simulink model "EcoSIM3_P2_C2_WIP"  (R2014b)
settings: Solver=ode1  SolverMode=SingleTasking  StartTime=0.0  StopTime=inf  FixedStep=0.01  RelTol=1e-3
PostLoadFcn:
  | %, if any(exist('dsrtsu_mdlpostloadfcn', 'file') == [2, 3, 6]), try dsrtsu_mdlpostloadfcn('Execute', bdroot); catch fprintf('Error in PostLoadFcn (dsrtsu_mdlpostloadfcn) for model "%s":\n %s\n', bdroot, lasterr); end, end,
InitFcn:
  | tic
  | %Startup_EcoSIM
values from neighbouring files (symbols this model uses):
  EngPwr = [0 5	10	15	20	25	30	35	40	45	50	55	60	65	70	75	80	85	90	95	100	105	110	115]    [Series_Maps.m]
  EngSpd = [0 477.4645 954.929 1909.858 2864.787 3819.716 4774.645 5729.574 6684.503]    [Series_Maps.m]
  EngTrq = [0	0	0	0	0	0	0	0	0	0	0	0	0	0	0	0	0	0	0	0	0	0	0	0 ... (first row only)    [Series_Maps.m]
  Power = [0 5 10 15 20 25 30]    [Series_Maps.m]
  Torque = [-50,-40,-30,-25,-20,-15,-10,-8,-6,-4,-2,0]    [Series_Maps.m]
undefined symbols (not defined in the file or in its folder): canChannel, Controls, DriveCycles, Driver, EM_EFF_MAP, EM_PwrLoss_MAP, Glbl, Overwritten_Mode, Plants, sigbuilder_block, Trialmap, Veh_Dynamics
libraries: simulink x141, canmsglib x113, fl_lib x104, canlib x89, nesl_utility x56, sdl_lib x29, dspsigops x6, dspswit3 x5, dspstat3 x2, commnoisgen2 x1, dspfdesign x1
(part 19 of 21)

== system EcoSIM3_P2_C2_WIP/Supervisory Controller/Functional Safety1/Functional Safety Algorithm/Fault Detection (Team Developed)/Torque Security Faults/Torque Estimation/Electric Motor Torque Estimation ==
  In1 : Inport
  Bus Selector : BusSelector  OutputSignals=Vehicle_Speed_meter_per_s,ESS_Transmit.bcm_vbat,ESS_Transmit.bcm_ibat,BAS_Transmit.BAS_Speed_rad_per_s,BAS_Transmit.BAS_Torque_Command_Nm
  EM DC Current Est : Subsystem
  EM Speed Est : Subsystem
  EM Torque Est : Subsystem
  Out1 : Outport
  wires:
  EM Torque Est/1(EM Trq Est [Nm]) -> Out1/1
  EM DC Current Est/1(EM DC Current Est [A]) -> EM Torque Est/3(EM DC Current Est [A])
  EM Speed Est/1(EM Speed Est [rad/s]) -> EM Torque Est/1(EM Speed [rad/s])
  Bus Selector/5 -> EM DC Current Est/4(BAS Torque [Nm])  "<BAS_Torque_Command_Nm>"
  Bus Selector/4 -> EM DC Current Est/3(BAS Speed [rad/s])  "<BAS_Speed_rad_per_s>"
  Bus Selector/3 -> EM DC Current Est/2(Batt Current [A])  "<bcm_ibat>"
  Bus Selector/2 -> EM Torque Est/2(Batt Voltage [V]), EM DC Current Est/1(Batt Voltage [V])  "<bcm_vbat>"
  Bus Selector/1 -> EM Speed Est/1(Vehicle Speed [m/s])  "<Vehicle_Speed_meter_per_s>"
  In1/1 -> Bus Selector/1

== system EcoSIM3_P2_C2_WIP/Supervisory Controller/Functional Safety1/Functional Safety Algorithm/Fault Detection (Team Developed)/Torque Security Faults/Torque Estimation/Engine Torque Estimation ==
  In1 : Inport
  Out1 : Outport

== system EcoSIM3_P2_C2_WIP/Supervisory Controller/Functional Safety1/Functional Safety Algorithm/Fault Detection (Team Developed)/Torque Security Faults/Torque Estimation/PTU Torque Estimation ==
  In1 : Inport
  Out1 : Outport

== system EcoSIM3_P2_C2_WIP/Supervisory Controller/Functional Safety1/Functional Safety Algorithm/Fault Detection (Team Developed)/Torque Security Faults/Torque Estimation/Rear Diff Torque Estimation ==
  In1 : Inport
  Out1 : Outport

== system EcoSIM3_P2_C2_WIP/Supervisory Controller/Functional Safety1/Functional Safety Algorithm/Fault Detection (Team Developed)/Torque Security Faults/Torque Estimation/Trans Torque Estimation ==
  In1 : Inport
  Out1 : Outport

== system EcoSIM3_P2_C2_WIP/Supervisory Controller/Functional Safety1/Functional Safety Algorithm/Fault Detection (Team Developed)/Torque Security Faults/Torque Estimation/Wheel Torque Estimation ==
  Veh Mass Est : Inport
  ECU/Sensor Signals : Inport  Port=2
  Bus Selector : BusSelector  OutputSignals=Vehicle_Speed_meter_per_s
  Derivative : Derivative
  Product : Product
  Product1 : Product
  Wheel Radius : Constant  Value=Plants.Rear_wh.tire_diameter/2
  Whl Trq Est : Outport
  wires:
  Bus Selector/1 -> Derivative/1  "<Vehicle_Speed_meter_per_s>"
  Derivative/1 -> Product/2  "Veh_Accel"
  Product1/1 -> Whl Trq Est/1  "Whl_Trq_Est_Nm"
  Wheel Radius/1 -> Product1/2
  Product/1 -> Product1/1
  ECU/Sensor Signals/1 -> Bus Selector/1
  Veh Mass Est/1 -> Product/1

== system EcoSIM3_P2_C2_WIP/Supervisory Controller/Functional Safety1/Functional Safety Algorithm/Fault Detection (Team Developed)/Torque Security Faults/Vehicle Mass Estimation/Belt Coupler ==
  BAS Torque : Inport
  Proportional Gain : Gain  Gain=Plants.Belt.GR
  Proportional Gain1 : Gain  Gain=Plants.Belt.GR
  Out1 : Outport
  wires:
  BAS Torque/1 -> Proportional Gain1/1
  Proportional Gain1/1 -> Proportional Gain/1
  Proportional Gain/1 -> Out1/1

== system EcoSIM3_P2_C2_WIP/Supervisory Controller/Functional Safety1/Functional Safety Algorithm/Fault Detection (Team Developed)/Torque Security Faults/Vehicle Mass Estimation/Driveline ==
  EM_Torque : Inport
  Mechanical Coupler : Subsystem
  Rear Diff : Subsystem
  Rear Wheels : Subsystem
  Out1 : Outport
  wires:
  Rear Wheels/1(Out1) -> Out1/1
  EM_Torque/1 -> Mechanical Coupler/1(In1)
  Mechanical Coupler/1(Out1) -> Rear Diff/1(In1)
  Rear Diff/1(Out1) -> Rear Wheels/1(In1)

== system EcoSIM3_P2_C2_WIP/Supervisory Controller/Functional Safety1/Functional Safety Algorithm/Fault Detection (Team Developed)/Torque Security Faults/Vehicle Mass Estimation/Driveline1 ==
  In1 : Inport
  Mechanical Coupler : Subsystem
  Rear Diff : Subsystem
  Rear Wheels : Subsystem
  Out1 : Outport
  wires:
  Rear Diff/1(Out1) -> Rear Wheels/1(In1)
  Mechanical Coupler/1(Out1) -> Rear Diff/1(In1)
  In1/1 -> Mechanical Coupler/1(In1)
  Rear Wheels/1(Out1) -> Out1/1

== system EcoSIM3_P2_C2_WIP/Supervisory Controller/Functional Safety1/Functional Safety Algorithm/Fault Detection (Team Developed)/Torque Security Faults/Vehicle Mass Estimation/Driveline2 ==
  In1 : Inport
  Mechanical Coupler : Subsystem
  Rear Diff : Subsystem
  Rear Wheels : Subsystem
  Out1 : Outport
  wires:
  Rear Wheels/1(Out1) -> Out1/1
  In1/1 -> Mechanical Coupler/1(In1)
  Mechanical Coupler/1(Out1) -> Rear Diff/1(In1)
  Rear Diff/1(Out1) -> Rear Wheels/1(In1)

== system EcoSIM3_P2_C2_WIP/Supervisory Controller/Functional Safety1/Functional Safety Algorithm/Fault Detection (Team Developed)/Torque Security Faults/Vehicle Mass Estimation/Resistance Forces ==
  Vehicle_Speed [m/s] : Inport
  Grade [%] : Inport  Port=2
  Vehicle_Mass [kg] : Inport  Port=3
  Aerodynamic Drag Function : Fcn  Expr=0.5*Glbl.den_air*Veh_Dynamics.Body.Aero_Drag_Coeff*Veh_Dynamics.Body.Frontal_Area*u^2
  Gain : Gain  Gain=Glbl.perc_to_frac
  Grade Resistance Function : Fcn  Expr=Glbl.g*sin(u)
  Percent Grade to Radians : Trigonometry  Operator=atan
  Product1 : Product  Inputs=**  RndMeth=Zero
  Rolling Resistance Function : Subsystem
  Sum1 : Sum  Inputs=+++  SaturateOnIntegerOverflow=on  InputSameDT=on  OutDataTypeStr=Inherit: Same as first input
  Road_Load_Force [N] : Outport
  wires:
  Grade [%]/1 -> Gain/1
  Gain/1 -> Percent Grade to Radians/1
  Vehicle_Mass [kg]/1 -> Product1/2, Rolling Resistance Function/1(Mass)
  Sum1/1 -> Road_Load_Force [N]/1  "Road_Load_Force_N"
  Vehicle_Speed [m/s]/1 -> Rolling Resistance Function/2(Vehicle Speed), Aerodynamic Drag Function/1
  Aerodynamic Drag Function/1 -> Sum1/1
  Grade Resistance Function/1 -> Product1/1
  Product1/1 -> Sum1/2
  Percent Grade to Radians/1 -> Rolling Resistance Function/3(Grade), Grade Resistance Function/1
  Rolling Resistance Function/1(Out2) -> Sum1/3

== system EcoSIM3_P2_C2_WIP/Supervisory Controller/Functional Safety1/Functional Safety Algorithm/Fault Detection (Team Developed)/Torque Security Faults/Vehicle Mass Estimation/Trans ==
  Current Gear : Inport
  ICE_Torque : Inport  Port=2
  Efficiency : Gain  Gain=Plants.Clutch.Eff
  Negative Torque : Gain  Gain=1/Plants.Trans.Mdl.Plant.eff  SaturateOnIntegerOverflow=on  OutDataTypeStr=Inherit: Same as input  ParamDataTypeStr=Inherit: Same as input
  Positive Torque : Gain  Gain=Plants.Trans.Mdl.Plant.eff  SaturateOnIntegerOverflow=on  OutDataTypeStr=Inherit: Same as input  ParamDataTypeStr=Inherit: Same as input
  Product1 : Product  SaturateOnIntegerOverflow=on  InputSameDT=on  OutDataTypeStr=Inherit: Same as first input
  Switch : Switch  SaturateOnIntegerOverflow=on  InputSameDT=on
  Trams GR : Lookup  InputValues=Plants.Trans.Mdl.Plant.Gear_cmd  Table=Plants.Trans.Mdl.Plant.GR  LookUpMeth=Use Input Nearest
  Out1 : Outport
  wires:
  Current Gear/1 -> Trams GR/1
  Switch/1 -> Out1/1  "Trans_Torque_Out_Nm"
  ICE_Torque/1 -> Efficiency/1
  Efficiency/1 -> Product1/2
  Product1/1 -> Switch/2, Positive Torque/1, Negative Torque/1
  Positive Torque/1 -> Switch/1
  Negative Torque/1 -> Switch/3
  Trams GR/1 -> Product1/1  "Trans_GR_Out"

== system EcoSIM3_P2_C2_WIP/Supervisory Controller/Functional Safety1/Functional Safety Algorithm/Fault Detection (Team Developed)/Torque Security Faults/Vehicle Mass Estimation/Trans1 ==
  Current Gear : Inport
  In1 : Inport  Port=2
  Efficiency : Gain  Gain=Plants.Clutch.Eff
  Negative Torque : Gain  Gain=1/Plants.Trans.Mdl.Plant.eff  SaturateOnIntegerOverflow=on  OutDataTypeStr=Inherit: Same as input  ParamDataTypeStr=Inherit: Same as input
  Positive Torque : Gain  Gain=Plants.Trans.Mdl.Plant.eff  SaturateOnIntegerOverflow=on  OutDataTypeStr=Inherit: Same as input  ParamDataTypeStr=Inherit: Same as input
  Product1 : Product  SaturateOnIntegerOverflow=on  InputSameDT=on  OutDataTypeStr=Inherit: Same as first input
  Switch : Switch  SaturateOnIntegerOverflow=on  InputSameDT=on
  Trams GR : Lookup  InputValues=Plants.Trans.Mdl.Plant.Gear_cmd  Table=Plants.Trans.Mdl.Plant.GR  LookUpMeth=Use Input Nearest
  Out1 : Outport
  wires:
  Trams GR/1 -> Product1/1  "Trans_GR_Out"
  Negative Torque/1 -> Switch/3
  Positive Torque/1 -> Switch/1
  Product1/1 -> Negative Torque/1, Positive Torque/1, Switch/2
  Efficiency/1 -> Product1/2
  In1/1 -> Efficiency/1
  Switch/1 -> Out1/1  "Trans_Torque_Out_Nm"
  Current Gear/1 -> Trams GR/1

== system EcoSIM3_P2_C2_WIP/Powertrain/Electrical Storage System/Soft ECU/Algorithm/Current Buffer/Charge Buffer/Moderator-Opposer/Moderator ==
  note: 0.061
  note: 0.1247
  I : Inport
  Compare To Constant : simulink/Logic and Bit Operations/Compare To Constant  relop=>=  const=50  OutDataTypeStr=boolean
  ModeratorHi : Gain  Gain=Plants.ESS.SoftECU.Buffer.Charge.ModeratorHi
  ModeratorLo : Gain  Gain=Plants.ESS.SoftECU.Buffer.Charge.ModeratorLo
  Switch : Switch  Criteria=u2 > Threshold  Threshold=0.5
  O : Outport
  wires:
  I/1 -> ModeratorHi/1, ModeratorLo/1
  ModeratorHi/1 -> Switch/1
  ModeratorLo/1 -> Switch/3
  Switch/1 -> O/1
  [Current] -> Compare To Constant/1
  Compare To Constant/1 -> Switch/2

== system EcoSIM3_P2_C2_WIP/Powertrain/Electrical Storage System/Soft ECU/Algorithm/Current Buffer/Charge Buffer/Moderator-Opposer/Opposer ==
  note: 0.4002
  note: 0.2799
  I : Inport
  Compare To Constant : simulink/Logic and Bit Operations/Compare To Constant  relop=>=  const=50  OutDataTypeStr=boolean
  OpposerHi : Gain  Gain=Plants.ESS.SoftECU.Buffer.Charge.OpposerHi
  OpposerLo : Gain  Gain=Plants.ESS.SoftECU.Buffer.Charge.OpposerLo
  Switch : Switch  Criteria=u2 > Threshold  Threshold=0.5
  O : Outport
  wires:
  [Current] -> Compare To Constant/1
  OpposerLo/1 -> Switch/3
  Compare To Constant/1 -> Switch/2
  OpposerHi/1 -> Switch/1
  Switch/1 -> O/1
  I/1 -> OpposerHi/1, OpposerLo/1

== system EcoSIM3_P2_C2_WIP/Powertrain/Electrical Storage System/Soft ECU/Algorithm/Current Buffer/Discharge Buffer/Moderator-Opposer/Moderator ==
  note: 0.0126
  note: 0.0319
  note: 0.0413
  note: Modeling discharge buffer- Approach 1
      | This model make the assumption that the current required to reduce the buffer is dependent on the current value of the buffer.
      | i.e the current required to cause a further reduction in the buffer when it is at 10% is greater than when it is at 90%. This model
      | multiplies the buffer spent (100- buffer) by a suitable gain (called the Opposer), subtracts it from the current provided by the battery,
      | and the difference is multiplied by a gain (called the Moderator) and integrated to change the buffer. The output of this integrator
      | can be considered as the buffer degradation. Subtracting this from 100 will give us the buffer.
      | Consider an initial buffer of 100%. If a constant current of 50 amps is provided by the battery, the buffer starts reducing, and then
      | reaches an equilibrium point. The buffer reduction rate is higher at the start, then starts reducing as the buffer drop. After reaching the
      | equilibrium point, the buffer remains constant when the current is kept constant. A further increase in current causes the buffer to drop,
      | while a lesser current causes the buffer to rise.
      | Also, it was observed from the dyno data that at a current < 130 amps, the buffer behaviour depends on the value of the current, while
      | at currents over 130 amps, the drop is independent of the current magnitude. Also, if the current exceeeds 340 amps, the buffer reduction
      | rate steepens.
      | Using the data from dyno testing, the Moderator and Opposer gains were calibrated, and the value of these gains was found for three
      | conditions-
      | a) Current < 130 amps (Buffer behaviour is dependent on current magnitude)
      | b) 130< Current < 340 amps (Buffer behaviour is independent of current magnitude)
      | c) Current >340 amps (Still independent, but fall is steeper than case 'b')
      |
      | It is assumed that if the current crosses 340 amps, it should go below 320 amps to begin using the gains from 'b' again. This lower
      | hysteresis value is yet to be verified.
  I : Inport
  Compare To Constant : simulink/Logic and Bit Operations/Compare To Constant  relop=>=  const=130  OutDataTypeStr=boolean
  ModeratorHi : Gain  Gain=Plants.ESS.SoftECU.Buffer.Discharge.ModeratorMax
  ModeratorHi1 : Gain  Gain=Plants.ESS.SoftECU.Buffer.Discharge.ModeratorHi
  ModeratorLo : Gain  Gain=Plants.ESS.SoftECU.Buffer.Discharge.ModeratorLo
  Relay : Relay  OnSwitchValue=340  OffSwitchValue=320
  Switch : Switch  Criteria=u2 > Threshold  Threshold=0.5
  Switch1 : Switch  Criteria=u2 > Threshold  Threshold=0.5
  O : Outport
  wires:
  I/1 -> ModeratorHi/1, ModeratorHi1/1, ModeratorLo/1
  ModeratorHi1/1 -> Switch1/3
  ModeratorLo/1 -> Switch/3
  Switch/1 -> O/1
  Compare To Constant/1 -> Switch/2
  ModeratorHi/1 -> Switch1/1
  [Current] -> Relay/1, Compare To Constant/1
  Relay/1 -> Switch1/2
  Switch1/1 -> Switch/1

== system EcoSIM3_P2_C2_WIP/Powertrain/Electrical Storage System/Soft ECU/Algorithm/Current Buffer/Discharge Buffer/Moderator-Opposer/Opposer ==
  note: -7.7656
  note: 1.0236
  note: 1.2456
  I : Inport
  Compare To Constant : simulink/Logic and Bit Operations/Compare To Constant  relop=>=  const=130  OutDataTypeStr=boolean
  OpposerHi : Gain  Gain=Plants.ESS.SoftECU.Buffer.Discharge.OpposerMax
  OpposerHi1 : Gain  Gain=Plants.ESS.SoftECU.Buffer.Discharge.OpposerHi
  OpposerLo : Gain  Gain=Plants.ESS.SoftECU.Buffer.Discharge.OpposerLo
  Relay : Relay  OnSwitchValue=340  OffSwitchValue=320
  Switch : Switch  Criteria=u2 > Threshold  Threshold=0.5
  Switch1 : Switch  Criteria=u2 > Threshold  Threshold=0.5
  O : Outport
  wires:
  [Current] -> Relay/1, Compare To Constant/1
  OpposerLo/1 -> Switch/3
  Compare To Constant/1 -> Switch/2
  Switch/1 -> O/1
  I/1 -> OpposerHi/1, OpposerHi1/1, OpposerLo/1
  Relay/1 -> Switch1/2
  OpposerHi/1 -> Switch1/1
  OpposerHi1/1 -> Switch1/3
  Switch1/1 -> Switch/1

== system EcoSIM3_P2_C2_WIP/Supervisory Controller/Functional Safety1/Functional Safety Algorithm/Fault Detection (Team Developed)/Torque Security Faults/Torque Comparisons/Electric Motor Torque Comparison/Faul_Detect ==
  Trq Est : Inport
  Trq feedback : Inport  Port=2
  Add : Sum
  Add1 : Sum  Inputs=+-
  Constant : Constant
  Logical Operator1 : Logic  Operator=OR  AllPortsSameDT=off  OutDataTypeStr=boolean
  Min Torque Threshold : Constant  Value=20
  Product : Product
  Product1 : Product
  Relational Operator : RelationalOperator  Operator=>  OutDataTypeStr=boolean
  Relational Operator2 : RelationalOperator  Operator=>  OutDataTypeStr=boolean
  Relational Operator3 : RelationalOperator  Operator=<  OutDataTypeStr=boolean
  Switch : Switch  Criteria=u2 > Threshold  Threshold=20
  Tolerance Determination (SS vs TRS) : Subsystem
  Trigger : Subsystem
  Fault : Outport
  wires:
  Constant/1 -> Add1/1, Add/1
  Add/1 -> Product/2  "Upper Limit"
  Add1/1 -> Product1/2  "Lower Limit"
  Relational Operator/1 -> Switch/3
  Min Torque Threshold/1 -> Relational Operator/2
  Logical Operator1/1 -> Switch/1
  Relational Operator2/1 -> Logical Operator1/1
  Relational Operator3/1 -> Logical Operator1/2
  Product/1 -> Relational Operator2/2
  Product1/1 -> Relational Operator3/2
  Trq Est/1 -> Tolerance Determination (SS vs TRS)/1(EM_TorqueOut_Est), Relational Operator/1, Switch/2, Product1/1, Product/1
  Tolerance Determination (SS vs TRS)/1(SS or Transient) -> Add/2, Add1/2
  Trq feedback/1 -> Relational Operator3/1, Relational Operator2/1
  Trigger/1(Out1) -> Fault/1
  Switch/1 -> Trigger/1(In1)

== system EcoSIM3_P2_C2_WIP/Supervisory Controller/Functional Safety1/Functional Safety Algorithm/Fault Detection (Team Developed)/Torque Security Faults/Torque Comparisons/Electric Motor Torque Comparison/Subsystem ==
  Trq Req : Inport
  Trq Est : Inport  Port=2
  Add : Sum
  Add1 : Sum  Inputs=-+
  Logical Operator1 : Logic  Operator=OR  AllPortsSameDT=off  OutDataTypeStr=boolean
  Relational Operator2 : RelationalOperator  Operator=>  OutDataTypeStr=boolean
  Relational Operator3 : RelationalOperator  Operator=<  OutDataTypeStr=boolean
  torque tolerance : Constant  Value=10
  Fault : Outport
  wires:
  torque tolerance/1 -> Add/1, Add1/1
  Trq Req/1 -> Add1/2, Add/2
  Relational Operator3/1 -> Logical Operator1/2
  Relational Operator2/1 -> Logical Operator1/1
  Add1/1 -> Relational Operator3/2
  Add/1 -> Relational Operator2/2
  Trq Est/1 -> Relational Operator2/1, Relational Operator3/1
  Logical Operator1/1 -> Fault/1

== system EcoSIM3_P2_C2_WIP/Supervisory Controller/Functional Safety1/Functional Safety Algorithm/Fault Detection (Team Developed)/Torque Security Faults/Torque Comparisons/Electric Motor Torque Comparison/Subsystem1 ==
  Trq Feedback : Inport
  Trq Req : Inport  Port=2
  Add : Sum
  Add1 : Sum  Inputs=-+
  Logical Operator : Logic  Operator=OR  AllPortsSameDT=off  OutDataTypeStr=boolean
  Relational Operator : RelationalOperator  Operator=>  OutDataTypeStr=boolean
  Relational Operator1 : RelationalOperator  Operator=<  OutDataTypeStr=boolean
  torque tolerance : Constant  Value=10
  Fault : Outport
  wires:
  torque tolerance/1 -> Add/1, Add1/1
  Add/1 -> Relational Operator/2
  Relational Operator/1 -> Logical Operator/1
  Trq Feedback/1 -> Relational Operator1/1, Relational Operator/1
  Logical Operator/1 -> Fault/1
  Trq Req/1 -> Add1/2, Add/2
  Add1/1 -> Relational Operator1/2
  Relational Operator1/1 -> Logical Operator/2

== system EcoSIM3_P2_C2_WIP/Supervisory Controller/Functional Safety1/Functional Safety Algorithm/Fault Detection (Team Developed)/Torque Security Faults/Torque Estimation/Electric Motor Torque Estimation/EM DC Current Est ==
  note: BAS HV current: need to update effeciency map to include inverter
      | DCDC HV current: need to update based on dbc files
      | HVAC current: ASSUME OFF, need to update
  Batt Voltage [V] : Inport
  Batt Current [A] : Inport  Port=2
  BAS Speed [rad/s] : Inport  Port=3
  BAS Torque [Nm] : Inport  Port=4
  Add : Sum  Inputs=++++
  Ask Shawn or Huster? : Constant  Value=2.8153
  BAS HV Current : Subsystem
  DCDC avg current [A] : Constant  Value=1.7918
  HVAC avg current [A] : Constant  Value=0
  Sum : Sum  Inputs=|+-
  EM DC Current Est [A] : Outport
  wires:
  Ask Shawn or Huster?/1 -> Add/4  "AccPwrMdlHiVltInpCrnt"
  BAS Torque [Nm]/1 -> BAS HV Current/3(BAS Torque [Nm])
  BAS HV Current/1(BAS DC Current [A]) -> Add/1
  BAS Speed [rad/s]/1 -> BAS HV Current/2(BAS Speed [rad/s])
  Sum/1 -> EM DC Current Est [A]/1  "EM_DC_Curent_Est_A"
  Add/1 -> Sum/2
  Batt Current [A]/1 -> Sum/1
  Batt Voltage [V]/1 -> BAS HV Current/1(Batt Voltage [V])
  HVAC avg current [A]/1 -> Add/3
  DCDC avg current [A]/1 -> Add/2

== system EcoSIM3_P2_C2_WIP/Supervisory Controller/Functional Safety1/Functional Safety Algorithm/Fault Detection (Team Developed)/Torque Security Faults/Torque Estimation/Electric Motor Torque Estimation/EM Speed Est ==
  note: update radius of wheels withe brielle info
  Vehicle Speed [m/s] : Inport
  Positive Torque : Gain  Gain=Plants.Rear_Diff.Diff_ratio  SaturateOnIntegerOverflow=on  OutDataTypeStr=Inherit: Same as input  ParamDataTypeStr=Inherit: Same as input
  Positive Torque1 : Gain  Gain=Plants.Mech_Coupler.EM_GR  SaturateOnIntegerOverflow=on  OutDataTypeStr=Inherit: Same as input  ParamDataTypeStr=Inherit: Same as input
  Positive Torque2 : Gain  Gain=2/(Plants.Front_wh.Tire.rollrad*2)  SaturateOnIntegerOverflow=on  OutDataTypeStr=Inherit: Same as input  ParamDataTypeStr=Inherit: Same as input
  EM Speed Est [rad/s] : Outport
  wires:
  Positive Torque1/1 -> EM Speed Est [rad/s]/1  "EM_Speed_Est_rad_per_s"
  Vehicle Speed [m/s]/1 -> Positive Torque2/1
  Positive Torque/1 -> Positive Torque1/1  "Shaft_Speed [rad/s]"
  Positive Torque2/1 -> Positive Torque/1  "Vehicle speed at wheels [rad/sec]"

== system EcoSIM3_P2_C2_WIP/Supervisory Controller/Functional Safety1/Functional Safety Algorithm/Fault Detection (Team Developed)/Torque Security Faults/Torque Estimation/Electric Motor Torque Estimation/EM Torque Est ==
  note: saturation: does not account for REGEN, aka negative current
  note: update based on plant models, which account for efficiency in torque!!
  EM Speed [rad/s] : Inport
  Batt Voltage [V] : Inport  Port=2
  EM DC Current Est [A] : Inport  Port=3
  Add : Sum  Inputs=-+
  Constant : Constant  Value=0
  Constant1 : Constant  Value=0
  EM + Inverter Eff Map : Lookup_n-D  Commented=on  BreakpointsForDimension1=EM_EFF_MAP.RPM  BreakpointsForDimension2=EM_EFF_MAP.TRQ  Table=EM_EFF_MAP.EFF  InternalRulePriority=Speed  RndMeth=Simplest  InputSameDT=on
  EM + Inverter Power Loss Map : Lookup_n-D  Commented=on  BreakpointsForDimension1=EM_PwrLoss_MAP.RPM  BreakpointsForDimension2=EM_PwrLoss_MAP.TRQ  Table=EM_PwrLoss_MAP.PWR_LOSS  InternalRulePriority=Speed  RndMeth=Simplest  InputSameDT=on
  EM Power Loss : Lookup2D  RowIndex=Plants.EM.Mdl.Plant.w_rad_PL  ColumnIndex=Plants.EM.Mdl.Plant.T_Nm_PL  Table=Plants.EM.Mdl.Plant.power_loss  LookUpMeth=Interpolation-Use End Values  SaturateOnIntegerOverflow=on  InputSameDT=on
  Gain : Gain
  Product : Product
  Product1 : Product  Inputs=/*
  Product2 : Product  Inputs=/*
  Saturation : Saturate  UpperLimit=inf  LowerLimit=0
  Switch : Switch  Criteria=u2 ~= 0
  Switch1 : Switch  Criteria=u2 ~= 0
  Terminator : Terminator
  EM Trq Est [Nm] : Outport
  wires:
  Constant1/1 -> Switch1/3
  Switch1/1 -> Terminator/1
  Product1/1 -> Switch/1
  Constant/1 -> Switch/3
  Product2/1 -> Switch1/1
  EM Power Loss/1 -> Add/1
  Add/1 -> Product2/2  "EM_Pwr_Out"
  Gain/1 -> EM Trq Est [Nm]/1  "EM_Trq_out_Est_Nm"
  Product/1 -> Product1/2, Add/2  "EM_Pwr_In_est_W"
  EM Speed [rad/s]/1 -> Product1/1, Switch/2, Switch1/2, Product2/1, EM Power Loss/1
  Switch/1 -> EM Power Loss/2, Gain/1  "EM_Trq_In_Est_Nm"
  Batt Voltage [V]/1 -> Product/1
  EM DC Current Est [A]/1 -> Saturation/1
  Saturation/1 -> Product/2

== system EcoSIM3_P2_C2_WIP/Supervisory Controller/Functional Safety1/Functional Safety Algorithm/Fault Detection (Team Developed)/Torque Security Faults/Vehicle Mass Estimation/Driveline/Mechanical Coupler ==
  In1 : Inport
  Differential Ratio2 : Constant  Value=Plants.Mech_Coupler.EM_GR
  Negative Torque : Gain  Gain=1/Plants.Mech_Coupler.EM_Eff  SaturateOnIntegerOverflow=on  OutDataTypeStr=Inherit: Same as input  ParamDataTypeStr=Inherit: Same as input
  Positive Torque : Gain  Gain=Plants.Mech_Coupler.EM_Eff  SaturateOnIntegerOverflow=on  OutDataTypeStr=Inherit: Same as input  ParamDataTypeStr=Inherit: Same as input
  Product2 : Product
  Switch1 : Switch  SaturateOnIntegerOverflow=on  InputSameDT=on
  Out1 : Outport
  wires:
  Differential Ratio2/1 -> Product2/2
  In1/1 -> Product2/1
  Switch1/1 -> Out1/1
  Positive Torque/1 -> Switch1/1
  Negative Torque/1 -> Switch1/3
  Product2/1 -> Switch1/2, Negative Torque/1, Positive Torque/1

== system EcoSIM3_P2_C2_WIP/Supervisory Controller/Functional Safety1/Functional Safety Algorithm/Fault Detection (Team Developed)/Torque Security Faults/Vehicle Mass Estimation/Driveline/Rear Diff ==
  In1 : Inport
  Differential Ratio2 : Constant  Value=Plants.Rear_Diff.Diff_ratio
  Divide : Product  Inputs=**
  Negative Torque : Gain  Gain=1/Plants.Rear_Diff.Eff  SaturateOnIntegerOverflow=on  OutDataTypeStr=Inherit: Same as input  ParamDataTypeStr=Inherit: Same as input
  Positive Torque : Gain  Gain=Plants.Rear_Diff.Eff  SaturateOnIntegerOverflow=on  OutDataTypeStr=Inherit: Same as input  ParamDataTypeStr=Inherit: Same as input
  Switch : Switch  SaturateOnIntegerOverflow=on  InputSameDT=on
  Out1 : Outport
  wires:
  Differential Ratio2/1 -> Divide/2
  Divide/1 -> Switch/2, Negative Torque/1, Positive Torque/1
  Switch/1 -> Out1/1
  Positive Torque/1 -> Switch/1
  In1/1 -> Divide/1
  Negative Torque/1 -> Switch/3

== system EcoSIM3_P2_C2_WIP/Supervisory Controller/Functional Safety1/Functional Safety Algorithm/Fault Detection (Team Developed)/Torque Security Faults/Vehicle Mass Estimation/Driveline/Rear Wheels ==
  In1 : Inport
  Divide : Product  Inputs=*/
  Wheel Radius : Constant  Value=Plants.Rear_wh.tire_diameter/2
  Out1 : Outport
  wires:
  In1/1 -> Divide/1
  Wheel Radius/1 -> Divide/2
  Divide/1 -> Out1/1

== system EcoSIM3_P2_C2_WIP/Supervisory Controller/Functional Safety1/Functional Safety Algorithm/Fault Detection (Team Developed)/Torque Security Faults/Vehicle Mass Estimation/Driveline1/Mechanical Coupler ==
  In1 : Inport
  Differential Ratio2 : Constant  Value=Plants.Mech_Coupler.EM_GR
  Negative Torque : Gain  Gain=1/Plants.Mech_Coupler.EM_Eff  SaturateOnIntegerOverflow=on  OutDataTypeStr=Inherit: Same as input  ParamDataTypeStr=Inherit: Same as input
  Positive Torque : Gain  Gain=Plants.Mech_Coupler.EM_Eff  SaturateOnIntegerOverflow=on  OutDataTypeStr=Inherit: Same as input  ParamDataTypeStr=Inherit: Same as input
  Product2 : Product
  Switch1 : Switch  SaturateOnIntegerOverflow=on  InputSameDT=on
  Out1 : Outport
  wires:
  Product2/1 -> Positive Torque/1, Negative Torque/1, Switch1/2
  Negative Torque/1 -> Switch1/3
  Positive Torque/1 -> Switch1/1
  Switch1/1 -> Out1/1
  In1/1 -> Product2/1
  Differential Ratio2/1 -> Product2/2

== system EcoSIM3_P2_C2_WIP/Supervisory Controller/Functional Safety1/Functional Safety Algorithm/Fault Detection (Team Developed)/Torque Security Faults/Vehicle Mass Estimation/Driveline1/Rear Diff ==
  In1 : Inport
  Differential Ratio2 : Constant  Value=Plants.Rear_Diff.Diff_ratio
  Divide : Product  Inputs=**
  Negative Torque : Gain  Gain=1/Plants.Rear_Diff.Eff  SaturateOnIntegerOverflow=on  OutDataTypeStr=Inherit: Same as input  ParamDataTypeStr=Inherit: Same as input
  Positive Torque : Gain  Gain=Plants.Rear_Diff.Eff  SaturateOnIntegerOverflow=on  OutDataTypeStr=Inherit: Same as input  ParamDataTypeStr=Inherit: Same as input
  Switch : Switch  SaturateOnIntegerOverflow=on  InputSameDT=on
  Out1 : Outport
  wires:
  Negative Torque/1 -> Switch/3
  In1/1 -> Divide/1
  Positive Torque/1 -> Switch/1
  Switch/1 -> Out1/1
  Divide/1 -> Positive Torque/1, Negative Torque/1, Switch/2
  Differential Ratio2/1 -> Divide/2

== system EcoSIM3_P2_C2_WIP/Supervisory Controller/Functional Safety1/Functional Safety Algorithm/Fault Detection (Team Developed)/Torque Security Faults/Vehicle Mass Estimation/Driveline1/Rear Wheels ==
  In1 : Inport
  Divide : Product  Inputs=*/
  Wheel Radius : Constant  Value=Plants.Rear_wh.tire_diameter/2
  Out1 : Outport
  wires:
  Divide/1 -> Out1/1
  Wheel Radius/1 -> Divide/2
  In1/1 -> Divide/1

== system EcoSIM3_P2_C2_WIP/Supervisory Controller/Functional Safety1/Functional Safety Algorithm/Fault Detection (Team Developed)/Torque Security Faults/Vehicle Mass Estimation/Driveline2/Mechanical Coupler ==
  In1 : Inport
  Differential Ratio2 : Constant  Value=Plants.Mech_Coupler.EM_GR
  Negative Torque : Gain  Gain=1/Plants.Mech_Coupler.EM_Eff  SaturateOnIntegerOverflow=on  OutDataTypeStr=Inherit: Same as input  ParamDataTypeStr=Inherit: Same as input
  Positive Torque : Gain  Gain=Plants.Mech_Coupler.EM_Eff  SaturateOnIntegerOverflow=on  OutDataTypeStr=Inherit: Same as input  ParamDataTypeStr=Inherit: Same as input
  Product2 : Product
  Switch1 : Switch  SaturateOnIntegerOverflow=on  InputSameDT=on
  Out1 : Outport
  wires:
  Differential Ratio2/1 -> Product2/2
  In1/1 -> Product2/1
  Switch1/1 -> Out1/1
  Positive Torque/1 -> Switch1/1
  Negative Torque/1 -> Switch1/3
  Product2/1 -> Switch1/2, Negative Torque/1, Positive Torque/1

== system EcoSIM3_P2_C2_WIP/Supervisory Controller/Functional Safety1/Functional Safety Algorithm/Fault Detection (Team Developed)/Torque Security Faults/Vehicle Mass Estimation/Driveline2/Rear Diff ==
  In1 : Inport
  Differential Ratio2 : Constant  Value=Plants.Rear_Diff.Diff_ratio
  Divide : Product  Inputs=**
  Negative Torque : Gain  Gain=1/Plants.Rear_Diff.Eff  SaturateOnIntegerOverflow=on  OutDataTypeStr=Inherit: Same as input  ParamDataTypeStr=Inherit: Same as input
  Positive Torque : Gain  Gain=Plants.Rear_Diff.Eff  SaturateOnIntegerOverflow=on  OutDataTypeStr=Inherit: Same as input  ParamDataTypeStr=Inherit: Same as input
  Switch : Switch  SaturateOnIntegerOverflow=on  InputSameDT=on
  Out1 : Outport
  wires:
  Differential Ratio2/1 -> Divide/2
  Divide/1 -> Switch/2, Negative Torque/1, Positive Torque/1
  Switch/1 -> Out1/1
  Positive Torque/1 -> Switch/1
  In1/1 -> Divide/1
  Negative Torque/1 -> Switch/3

== system EcoSIM3_P2_C2_WIP/Supervisory Controller/Functional Safety1/Functional Safety Algorithm/Fault Detection (Team Developed)/Torque Security Faults/Vehicle Mass Estimation/Driveline2/Rear Wheels ==
  In1 : Inport
  Divide : Product  Inputs=*/
  Wheel Radius : Constant  Value=Plants.Rear_wh.tire_diameter/2
  Out1 : Outport
  wires:
  In1/1 -> Divide/1
  Wheel Radius/1 -> Divide/2
  Divide/1 -> Out1/1

== system EcoSIM3_P2_C2_WIP/Supervisory Controller/Functional Safety1/Functional Safety Algorithm/Fault Detection (Team Developed)/Torque Security Faults/Vehicle Mass Estimation/Resistance Forces/Rolling Resistance Function ==
  Mass : Inport
  Vehicle Speed : Inport  Port=2
  Grade : Inport  Port=3
  Bias : Bias  Bias=Veh_Dynamics.Res_Forces.C_roll_res
  Constant1 : Constant  Value=Veh_Dynamics.Res_Forces.Const1
  Fcn : Fcn  Expr=u(2)*(2-tanh(5*(u(1)-2)))
  Gain1 : Gain  Gain=Veh_Dynamics.Res_Forces.Gain1
  Math Function : Math  Operator=pow  SaturateOnIntegerOverflow=on
  Mux : Mux  Inputs=2
  Mux1 : Mux  Inputs=2
  Product2 : Product  Inputs=**  RndMeth=Zero
  Rolling Resistance Function : Fcn  Expr=Glbl.g*u(1)*cos(u(2))
  Out2 : Outport
  wires:
  Fcn/1 -> Out2/1
  Grade/1 -> Mux/2
  Vehicle Speed/1 -> Mux1/1, Math Function/1
  Mass/1 -> Product2/2
  Product2/1 -> Mux1/2
  Rolling Resistance Function/1 -> Product2/1
  Constant1/1 -> Math Function/2
  Mux/1 -> Rolling Resistance Function/1
  Math Function/1 -> Gain1/1
  Bias/1 -> Mux/1
  Gain1/1 -> Bias/1
  Mux1/1 -> Fcn/1

== system EcoSIM3_P2_C2_WIP/Supervisory Controller/Functional Safety1/Functional Safety Algorithm/Fault Detection (Team Developed)/Torque Security Faults/Torque Comparisons/Electric Motor Torque Comparison/Faul_Detect/Tolerance Determination (SS vs TRS) ==
  EM_TorqueOut_Est : Inport
  Abs : Abs
  Add2 : Sum  Inputs=+-
  Constant1 : Constant  Value=2
  Relational Operator1 : RelationalOperator  Operator=<=  OutDataTypeStr=boolean
  SS Tolerance : Constant  Value=.1
  Switch1 : Switch  Criteria=u2 > Threshold  Threshold=.5
  Transfer Fcn : TransferFcn  Denominator=[.025 1]
  Transfer Fcn1 : TransferFcn  Denominator=[.025 1]
  Transient Tolerance : Constant  Value=.2
  Transport Delay : TransportDelay  DelayTime=.02
  SS or Transient : Outport
  wires:
  Transport Delay/1 -> Transfer Fcn1/1
  Transfer Fcn/1 -> Add2/1
  Transfer Fcn1/1 -> Add2/2
  Add2/1 -> Abs/1
  Abs/1 -> Relational Operator1/1  "transient_determination"
  Constant1/1 -> Relational Operator1/2
  Switch1/1 -> SS or Transient/1  "TM_Torque_Est_Tolerance"
  Relational Operator1/1 -> Switch1/2
  SS Tolerance/1 -> Switch1/1
  EM_TorqueOut_Est/1 -> Transfer Fcn/1, Transport Delay/1
  Transient Tolerance/1 -> Switch1/3

== system EcoSIM3_P2_C2_WIP/Supervisory Controller/Functional Safety1/Functional Safety Algorithm/Fault Detection (Team Developed)/Torque Security Faults/Torque Comparisons/Electric Motor Torque Comparison/Faul_Detect/Trigger ==
  In1 : Inport
  Constant : Constant  Value=-.01
  Data Type Conversion1 : DataTypeConversion
  Gain : Gain  Gain=10
  Integrator1 : Integrator  LimitOutput=on  UpperSaturationLimit=1  LowerSaturationLimit=0
  Sum : Sum  Inputs=+-
  Trigger Threshold : simulink/Logic and Bit Operations/Compare To Constant  relop=>=  const=1  OutDataTypeStr=boolean
  Out1 : Outport
  wires:
  Integrator1/1 -> Trigger Threshold/1
  Trigger Threshold/1 -> Out1/1
  In1/1 -> Data Type Conversion1/1
  Constant/1 -> Sum/2
  Data Type Conversion1/1 -> Sum/1
  Sum/1 -> Gain/1
  Gain/1 -> Integrator1/1

== system EcoSIM3_P2_C2_WIP/Supervisory Controller/Functional Safety1/Functional Safety Algorithm/Fault Detection (Team Developed)/Torque Security Faults/Torque Estimation/Electric Motor Torque Estimation/EM DC Current Est/BAS HV Current ==
  Batt Voltage [V] : Inport
  BAS Speed [rad/s] : Inport  Port=2
  BAS Torque [Nm] : Inport  Port=3
  BAS efficiency map : Lookup_n-D  BreakpointsForDimension1=Plants.BAS.Mdl.Plant.N_RPM  BreakpointsForDimension2=Plants.BAS.Mdl.Plant.T_Nm  Table=Plants.BAS.Mdl.Plant.Eff  InternalRulePriority=Speed  RndMeth=Simplest  InputSameDT=on
  Product : Product
  Product1 : Product  Inputs=*/
  Product2 : Product  Inputs=/*
  rad/s to rpm : Gain  Gain=30/pi
  to percent : Gain  Gain=.01
  BAS DC Current [A] : Outport
  wires:
  Product/1 -> Product1/1  "BAS_Pwer_Out_W"
  Product2/1 -> BAS DC Current [A]/1  "BAS_Current_A"
  Product1/1 -> Product2/2  "BAS_Pwer_In_W"
  Batt Voltage [V]/1 -> Product2/1
  BAS efficiency map/1 -> to percent/1
  rad/s to rpm/1 -> BAS efficiency map/1
  to percent/1 -> Product1/2
  BAS Torque [Nm]/1 -> Product/2, BAS efficiency map/2
  BAS Speed [rad/s]/1 -> Product/1, rad/s to rpm/1

== stateflow chart EcoSIM3_P2_C2_WIP/Supervisory Controller/Mode Operation/Limited EV/Temperature Limiting Disbuf/Chart ==
  state EM
    entry: out=1
  state Normal
    entry: out=4;
  state Inverter
    entry: out=2
  state Battery
    entry: out=3
  Normal -> EM [order 1] : [EM>100]
  (default) -> Normal
  Normal -> Inverter [order 2] : [Inverter>70]
  Normal -> Battery [order 3] : [ESS_discharge_buffer<=0.9]
  data: EM input; Inverter input; ESS_discharge_buffer input; out output

== stateflow chart EcoSIM3_P2_C2_WIP/Powertrain/Electrical Storage System/Soft ECU/Algorithm/A123 BMS ==
  state ChargeOver
    entry: bcm_chgc_stat=0;
    chga_ena=0;
    bcm_on_plug=0;
    bcm_ready=0;
  note: Do we put Veh_wake in here? Where is it connected in the vehicle?
  state ChargingMode
    entry: bcm_chgc_stat=1;
    chga_ena=1;
    bcm_on_plug=1;
    bcm_ready=1;
  state StartVehicleMonitoring
    bcm_ready=0;
    bcm_hvil_mon=0;
    bcm_mainc_stat=0;
    bcm_chgc_stat=0;
    bcm_cpwr_cmd=0;
    bcm_cpwr_mon=0;
    bcm_epo=0;
    bcm_veh_mon=1;
  state Startup
    bcm_ready=0;
    bcm_hvil_mon=1;
    bcm_mainc_stat=0;
    bcm_chgc_stat=0;
    bcm_cpwr_cmd=0;
    bcm_cpwr_mon=0;
    bcm_epo=0;
  state WaitforPowerUp
  state Operation
    state Wait_for_enable
      bcm_ready=1;
      bcm_hvil_mon=1;
      bcm_mainc_stat=0;
      bcm_chgc_stat=0;
      bcm_cpwr_cmd=0;
      bcm_cpwr_mon=0;
      bcm_epo=0;
    state Wait_for_mainc_close
      bcm_ready=1;
      bcm_hvil_mon=1;
      bcm_mainc_stat=0;
      bcm_chgc_stat=0;
      bcm_cpwr_cmd=1;
      bcm_cpwr_mon=1;
      bcm_epo=0;
    state Contactors_closed
      bcm_ready=1;
      bcm_hvil_mon=1;
      bcm_mainc_stat=1;
      bcm_chgc_stat=0;
      bcm_cpwr_cmd=1;
      bcm_cpwr_mon=1;
      bcm_epo=0;
    Wait_for_enable -> Wait_for_mainc_close : [hsc_bcm_enable==1]
    Wait_for_mainc_close -> Contactors_closed [order 2] : [hsc_bcm_mainc_close==1]
    (default) -> Wait_for_enable
    Wait_for_mainc_close -> Wait_for_enable [order 1] : [hsc_bcm_enable==0]
    Contactors_closed -> Wait_for_mainc_close : [hsc_bcm_mainc_close==0]
  state ReadyToCharge
    entry: bcm_chgc_stat=0;
    chga_ena=1;
    bcm_on_plug=1;
    bcm_ready=1;
  state WaitforLeakageEnable
    entry: bcm_chgc_stat=0;
    chga_ena=0;
    bcm_on_plug=0;
  state Fault
    bcm_ready=0;
    bcm_hvil_mon=1;
    bcm_mainc_stat=0;
    bcm_chgc_stat=0;
    bcm_cpwr_cmd=0;
    bcm_cpwr_mon=0;
    bcm_epo=1;
  state Shutdown
    bcm_ready=0;
    bcm_hvil_mon=0;
    bcm_mainc_stat=0;
    bcm_chgc_stat=0;
    bcm_cpwr_cmd=0;
    bcm_cpwr_mon=0;
    bcm_epo=0;
    bcm_veh_mon=0;
  ChargingMode -> ChargeOver : [chga_wake==0]
  ChargeOver -> WaitforPowerUp
  (default) -> WaitforPowerUp
  ReadyToCharge -> ChargingMode : [Charger_On==1]
  Startup -> Operation [order 1] : [hsc_bcm_enable==0]
  WaitforPowerUp -> WaitforLeakageEnable : [PowerUp==1]
  WaitforLeakageEnable -> ReadyToCharge [order 1] : [chga_wake==1]
  WaitforLeakageEnable -> StartVehicleMonitoring [order 2] : [hsc_bcm_leakage_ena==1 ...
      | && veh_wake==1]
  StartVehicleMonitoring -> Startup
  Shutdown -> WaitforLeakageEnable
  Startup -> Fault [order 2] : [hsc_bcm_enable==1|| hsc_bcm_epo==1]
  Operation -> Shutdown [order 2] : [veh_wake ==0]
  Operation -> Fault [order 1] : [bcm_cell_temp < bcm_cell_t_lower_lim || ...
      |  bcm_cell_temp > bcm_cell_t_upper_lim ||...
      | bcm_dis_buffer < 5 || hsc_bcm_epo==1]
  data: PowerUp input double; hsc_bcm_enable input double; hsc_bcm_mainc_close input double; bcm_ready output double; bcm_hvil_mon output double; bcm_mainc_stat output double; bcm_chgc_stat output double; bcm_cpwr_cmd output double; bcm_cpwr_mon output double; bcm_epo output double; bcm_cell_temp input double; hsc_bcm_epo input double; hsc_bcm_leakage_ena input double; veh_wake input double; chga_wake input double; bcm_dis_buffer input double; bcm_veh_mon output double; bcm_cell_t_upper_lim input double; bcm_cell_t_lower_lim input double; chga_ena output double; bcm_on_plug output double; Charger_On input double

== stateflow chart EcoSIM3_P2_C2_WIP/Driver/Startup Dummy/Vehicle Start/Chart1 ==
  state Entry
    entry: Key_State=0;
    SysPwrMd=0;
  state entry3
    entry: Key_State=1;
    SysPwrMd=2;
  state State1
    entry: Key_State=1;
    SysPwrMd=1;
  state entry2
    entry: Key_State=0;
    SysPwrMd=0;
  state entry4
    entry: Key_State=1;
    SysPwrMd=2;
  state entry1
    entry: Key_State=1;
    SysPwrMd=1;
  (default) -> Entry
  entry2 -> Entry : [Push_Button==0]
  Entry -> entry3 [order 2] : [Push_Button==1 &&...
      | Brk_PRNDL==1]
  Entry -> State1 [order 1] : [Push_Button==1&&...
      | Brk_PRNDL==0]
  entry1 -> entry3 [order 2] : [Push_Button==1 &&...
      | Brk_PRNDL==1]
  entry3 -> entry4 : [Push_Button==0]
  entry4 -> entry2 : [Push_Button==1]
  State1 -> entry1 : [Push_Button==0]
  entry1 -> entry2 [order 1] : [Push_Button==1 &&...
      | Brk_PRNDL==0]
  data: Push_Button input; Brk_PRNDL input; Key_State output; SysPwrMd output

== stateflow chart EcoSIM3_P2_C2_WIP/Driver/Startup Dummy/Vehicle Start/Park_check ==
  state Park
    en, du: position = 1;
  state NotPark
    en, du: position = p_in;
  (default) -> Park
  NotPark -> Park : [beta >= 20 && p_in == 1]
  Park -> NotPark : [beta >= 20 && p_in ~= 1]
  data: p_in input; beta input; position output

== stateflow chart EcoSIM3_P2_C2_WIP/Supervisory Controller/Mode Operation/Charging/ESS_Messages/ESS Handshake ==
  note: The ESS handshake ensures that the hsc_bcm_enable signal commands is sent by the supervisory only when the bcm is in the appropriate readiness state
  state Entry
    entry: hsc_bcm_enable=0;
    en: hsc_bcm_leakage_ena=1;
    en: hsc_bcm_mainc_close=0;
  state WaitforBCMReady
  state Enable
    entry: hsc_bcm_enable=1;
    during: hsc_bcm_enable=1;
  state CloseContactors
    entry:hsc_bcm_mainc_close=1;
    during:hsc_bcm_mainc_close=1;
    during:hsc_bcm_enable=1;
  (default) -> Entry
  Entry -> WaitforBCMReady : [bcm_veh_mon==1 && Veh_Start==1]
  WaitforBCMReady -> Enable : [bcm_ready==1]
  Enable -> CloseContactors : [bcm_cpwr_cmd==1 && bcm_cpwr_mon==1]
  data: bcm_ready input double; bcm_cpwr_cmd input double; bcm_cpwr_mon input double; hsc_bcm_enable output double; hsc_bcm_mainc_close output double; hsc_bcm_leakage_ena output; bcm_veh_mon input; bcm_mainc_stat input; Veh_Start input double

== stateflow chart EcoSIM3_P2_C2_WIP/Powertrain/Accessories Power Module/Component Power/HVAC/HVAC softECU ==
  state Entry
    entry: Compressor_status=0;
    entry: Compressor_speed_rpm=0;
  state Operation
    state CompOff
      entry: Compressor_status=0;
      entry: Compressor_speed_rpm=0;
    state CompOn
      entry: Compressor_status=1;
      entry: Compressor_speed_rpm=1500;
    (default) -> CompOff
    CompOff -> CompOn : [AC_Press_bar< ...
        | AC_engagement_pressure]
    CompOn -> CompOff : [AC_Press_bar > AC_max_pressure]
  (default) -> Entry
  Operation -> Entry : [AC_Mode==0]
  Entry -> Operation : [AC_Mode==1]
  data: AC_Mode input; AC_Press_bar input; AC_engagement_pressure input; AC_max_pressure input; Compressor_status output; Compressor_speed_rpm local

== stateflow chart EcoSIM3_P2_C2_WIP/Driver/Startup Dummy/Chart ==
  state Wait1
  state Zero
    entry: output=0;
  state One
    entry: output=1;
  state Wait
  (default) -> Zero
  Zero -> Wait1 : [input==0]
  Wait -> Zero : [input==1]
  Wait1 -> One : [input==1]
  One -> Wait : [input==0]
  data: input input; output output

== stateflow chart EcoSIM3_P2_C2_WIP/Powertrain/Clutch_Transmission2/CP1 SoftEcu/Algorithm/Chart ==
  note: Clutch_Sw - 0= Clutch fully engaged
      |                        1= Clutch fully disengaged (Pedal completely pressed
      |                        2= Engagement/ Disengagement in process (This state has been introduced so that Mastershift does not shift
      | accidentally while clutch is being engaged, and GCM does not allow torque transmission before clutch is fully engaged
      |
      | Clutch_Request- Request to press (disengage) the clutch
      | 0= Engage the clutch  (Foot off the pedal)
      | 1= Disengage the clutch (Press the pedal)
  state SecureMode
    entry: Mode=1;
    Position_Command=0;
  state Init
    entry: Mode=0;
  state OperationMode
    entry: Mode=2;
    en,du: Position_Command=Position_Request;
  (default) -> Init
  Init -> SecureMode
  SecureMode -> OperationMode
  data: Position_Command output; Position_Request input; Mode output

== stateflow chart EcoSIM3_P2_C2_WIP/Powertrain/Clutch_Transmission2/Mastershift Softecu/Algorithm/Chart ==
  note: Do we implement the clutch timeout as given in Mastershift doc?
      | We won't need it because supervisory will always give clutch request
      | along with gear request
  state ResetCounter
    entry: reset=-5;
  note: Time period taken into consideration to count the
      | no. of Upshifts/ Downshifts
  state Comeon
    entry: reset=0;
    entry: Local_Count=Count;
    entry: Gear_Cmd=Actual_Gear;
    entry: TCM_Gear=Actual_Gear;
  state Start
    entry: Local_Count=Count;
    entry:reset=0;
    during: Local_Count=Count;
  state CounterReset
    entry: reset=1;
  state StartShifting
    entry: Gear_Cmd=Actual_Gear+round(Local_Count);
    during: Gear_Cmd=Actual_Gear+round(Local_Count);
  note: Currently, the softecu directly receives the Gear requested by the GCM and proceeds to shift into that gear when
      | the clutch is pressed.
      | The final softecu is supposed to receive 'Upshift' and 'Downshift' commands from the GCM in the form of blips.
      | It will then count the number of blips and add it to the existing gear, effectively counting the gear requested.
      | The timeout state is set so that if the softecu does not receive confirmation that the clutch is disengaged some time
      | after the gear change request is received, it will not shift. The timeout values are generally between (3000 ms and 5000 ms)
      | according the Mastershift documentation. We probably won't require the timeout function in the softecu because the GCM
      | should take care of the clutch command.
      | This stateflow now loops between Default and Timeout Wait if the ClutchSw~=1 and Gear Requested is kept the same. The
      | cancelling of the original gear request can be implemented using the reset counter once the Upshift/Downshift is completed
  state ShiftingComplete
    entry: TCM_Gear=Actual_Gear;
    entry: reset=-5; %Counter has rising edge trigger
    during: TCM_Gear=Actual_Gear;
    during: Local_Count=Count;
  ResetCounter -> Start
  StartShifting -> ResetCounter [order 2] : [Gear_Cmd>5||Gear_Cmd<-1]
  (default) -> Comeon
  Start -> CounterReset : [Clutch_Sw==1]
  Comeon -> Start : [Count~=0]
  CounterReset -> StartShifting
  ShiftingComplete -> Comeon : [Clutch_Sw==0]
  StartShifting -> ShiftingComplete [order 1] : [Actual_Gear==Gear_Cmd]
  data: Clutch_Sw input; Actual_Gear input; Gear_Cmd output; TCM_Gear output; reset output; Local_Count local; Count input

== stateflow chart EcoSIM3_P2_C2_WIP/Powertrain/Charger/Soft ECU/Algorithm/Chart ==
  state Entry
    entry: chga_wake=0;
    GCM_Wakeup_charge=0;
    charge_start=0;
  state Charge
    entry: chga_wake=1;
    GCM_Wakeup_charge=1;
    charge_start=0;
  state ChargeEnabled
    entry: chga_wake=1;
    GCM_Wakeup_charge=1;
    charge_start=1;
  (default) -> Entry
  Charge -> Entry [order 1] : [AC_Supply==0]
  ChargeEnabled -> Entry : [AC_Supply==0||PON==0]
  Entry -> Charge : [AC_Supply==1]
  Charge -> ChargeEnabled [order 2] : [PON==1]
  data: AC_Supply input; chga_wake output; GCM_Wakeup_charge output; PON input; charge_start output

== stateflow chart EcoSIM3_P2_C2_WIP/Powertrain/BAS Motor/Soft ECU/Algorithm/BAS Stateflow ==
  note: Mode Request is similar to Inverter Enable / Disable
  state StartupShutdownSequence [group]
    state StartState
      during: Commanded_Torque = 0;
      %Loading EEPROM Parameters & carrying out POST (Power On Self Tests)
    state Standby
      % Entry point into Inverter
      % State Machine
    state Startup_Sequence
      state Inverter_Wait
        entry: FaultState=0;
        during: Commanded_Torque =0;
      state Inverter_Ready
        during: Commanded_Torque =0;
        entry: InverterStatusMode = 1;
        during: InverterStatusMode = 1;
      Inverter_Wait -> Inverter_Ready : [ModeRequest >= 1]
    state Torque_Control_Mode
      state SpeedGreaterThanMaxSpeed
        entry: Commanded_Torque=0;
        during: Commanded_Torque = 0;
      state ValidSpeed
        entry: Commanded_Torque=Torque_Command;
        during: Commanded_Torque=Torque_Command;
      state SpeedGreaterThanMaxSpeed1 [commented out]
        entry: Commanded_Torque=0;
      (default) -> (junction 53)
      (junction 53) -> SpeedGreaterThanMaxSpeed [order 1] : [abs (MotorSpeed) > MotorMaxSpeed]
      (junction 53) -> (junction 60) [order 2]
      SpeedGreaterThanMaxSpeed -> (junction 60) : [abs (MotorSpeed) <= MotorMaxSpeed]
      (junction 60) -> ValidSpeed
      ValidSpeed -> SpeedGreaterThanMaxSpeed [commented out] : [abs (MotorSpeed) > MotorMaxSpeed]
      ValidSpeed -> SpeedGreaterThanMaxSpeed1 [commented out] : [MotorSpeed<= 83*BeltRatio]
      SpeedGreaterThanMaxSpeed1 -> ValidSpeed [commented out] : [MotorSpeed>84*BeltRatio]
    state ShutdownInProcess
    state FaultState
      entry: FaultState = 1;
      during: FaultState = 1;
      % to exit this state, power must be cycled
    (default) -> Standby
    Standby -> StartState : [Power_up == 1 && ...
        | POST_Fault == 0 ]
    StartState -> FaultState [order 2] : [Power_up == 1 ...
        | &&POST_Fault == 1]
    StartState -> Inverter_Wait [order 1] : [Power_up == 1 ...
        | &&POST_Fault == 0]
    ShutdownInProcess -> Standby : [Power_up == 0]
    (junction 28) -> ShutdownInProcess [order 2] : [Power_up ==0]
    FaultState -> ShutdownInProcess : [Power_up == 0 ]
    Inverter_Ready -> Torque_Control_Mode : [MotorFault==0]
    (junction 28) -> FaultState [order 1] : [MotorFault ==1]
    Torque_Control_Mode -> (junction 28) : [MotorFault==1]
  data: MotorSpeed input; Power_up input; ModeRequest input; Torque_Command input; MotorMaxSpeed input; POST_Fault input; BeltRatio input; MotorFault input; Commanded_Torque output; InverterStatusMode output; FaultState output
